simulink model "nav_flocking33"  (R2022b)
settings: Solver=FixedStepAuto  StartTime=0.0  StopTime=10.0  FixedStep=0.01  RelTol=1e-3
values from neighbouring files (symbols this model uses):
  a = 1    [main_flock3.m]    (also in main_flock4.m; params_flocking_ros.m)
  aR = diag([ar; ap; ay])    [main_flock3.m]    (also in main_flock4.m; main_sliding.m)
  Att1 = [2 -2 -15]    [main_flock3.m]    (also in main_flock4.m)
  Att2 = [2 -2 -15]    [main_flock3.m]    (also in main_flock4.m)
  Att3 = [2 -2 -15]    [main_flock3.m]    (also in main_flock4.m)
  b = 1    [main_flock3.m]    (also in main_flock4.m; params_flocking_ros.m)
  c = 1    [main_flock3.m]    (also in main_flock4.m; params_flocking_ros.m)
  c_gammap = 1.2    [main_flock3.m]    (also in main_flock4.m)
  c_gammav = 3.5    [main_flock3.m]    (also in main_flock4.m)
  d = 0.6    [main_flock3.m]    (also in main_flock4.m; params_flocking_ros.m)
  d_prime = 1    [main_flock3.m]    (also in main_flock4.m; params_flocking_ros.m)
  epsilon = 0.1    [main_flock3.m]    (also in main_flock4.m; params_flocking_ros.m)
  h = 0.2    [main_flock3.m]    (also in main_flock4.m; params_flocking_ros.m)
  K1 = diag([k111; k122; k133])    [main_flock3.m]    (also in main_flock4.m; main_sliding.m)
  K2 = diag([k211; k222; k233])    [main_flock3.m]    (also in main_flock4.m; main_sliding.m)
  Ki = diag([Ki1; Ki2; Ki3])    [main_flock3.m]    (also in main_flock4.m; main_sliding.m)
  lam = diag([lam1; lam2; lam3])    [main_flock3.m]    (also in main_flock4.m; main_sliding.m)
  R = 0.15    [main_flock3.m]    (also in main_flock4.m; params_flocking_ros.m)
  vxobs = 0    [main_flock3.m]    (also in main_flock4.m)
  vyobs = 0    [main_flock3.m]    (also in main_flock4.m)
  vzobs = 0    [main_flock3.m]    (also in main_flock4.m)
  X0_1 = [P01 dP01 om01]    [main_flock3.m]    (also in main_flock4.m; main_sliding.m = [P0 dP0 om0])
  X0_2 = [P02 dP02 om02]    [main_flock3.m]    (also in main_flock4.m)
  X0_3 = [P03 dP03 om03]    [main_flock3.m]    (also in main_flock4.m)
  xmax = 2    [main_flock3.m]    (also in main_flock4.m)
  xmin = -2    [main_flock3.m]    (also in main_flock4.m)
  xobs = 0.75    [main_flock3.m]    (also in main_flock4.m)
  yobs = -0.25    [main_flock3.m]    (also in main_flock4.m)
  zobs = 1.7    [main_flock3.m]    (also in main_flock4.m)
undefined symbols (not defined in the file or in its folder): A_Euler
libraries: aerosimlib x3
(part 2 of 2)

== matlab function nav_flocking33/Dron_dynamics2/Mixer (Parrot ARDRONE) ==
  data: T input; w1 output size=1; tau input; w2 output size=1; w3 output size=1; w4 output size=1
function [w1,w2,w3,w4]   = fcn(T, tau)
%#codegen
tau_phi = tau(1); 
tau_the = tau(2); 
tau_psi = tau(3);

% This values vary in fonction of the geometry of the drone 
b= 4.06e-6;
d= 7.5e-7;
l= (0.2)*(sin(pi/4));

%Parrot AR-DRONE 
uT = T/b; 
uphi = (sqrt(2)*tau_phi)/(b*l);  
uthe = (sqrt(2)*tau_the)/(b*l);
upsi = tau_psi/(d*l);

%Mix by Motors
mixM1 = uT+uphi-uthe+upsi;  %uT + for all mixM
mixM2 = uT-uphi-uthe-upsi; 
mixM3 = uT-uphi+uthe+upsi; 
mixM4 = uT+uphi+uthe-upsi;

%rotors speeds [rads/s]
w1= sign(mixM1)*sqrt(abs((1/4)*mixM1));
w2= sign(mixM2)*sqrt(abs((1/4)*mixM2));
w3= sign(mixM3)*sqrt(abs((1/4)*mixM3));
w4= sign(mixM4)*sqrt(abs((1/4)*mixM4));

== matlab function nav_flocking33/Subsystem2/Sliding mode (quaternions) ==
  data: qwe input; Gamma output; lam parameter; Ki parameter; K1 parameter; K2 parameter; aR parameter; s output
function [Gamma, s]  = fcn(qwe, lam, Ki, K1, K2, aR)

%Rotorcraft dimensions and parameters
Ix = 7.5e-3;
Iy = 7.5e-3;
Iz = 1.3e-2;

%Inertia
Ii=[Ix 0 0; 0 Iy 0; 0 0 Iz];

%Separation of rotational velocity and quaternion error in its components
qe = qwe(5:8);
qe1 = qe(1);
qe2 = qe(2);
qe3 = qe(3);
qe4 = qe(4);
qev = [qe2; qe3; qe4];

w = qwe(9:11);

iqe = qwe(12:15);
i_qe = [iqe(2); iqe(3); iqe(4)];

%Desired rotational velocity
wd = [0;0;0];

dwd = [0;0;0];

%Rotational velocity error in Euler
we = w - wd;
we1 = we(1);
we2 = we(2);
we3 = we(3);

%Quaternion error (derivative)
dqe0 = 0.5*(-we1*qe2 - we2*qe3 - we3*qe4);
dqe1 = 0.5*(we1*qe1 + we3*qe3 - we2*qe4);
dqe2 = 0.5*(we2*qe1 - we3*qe2 + we1*qe4);
dqe3 = 0.5*(we3*qe1 + we2*qe2 - we1*qe3);
dqe = [dqe1; dqe2; dqe3];

%Identity matrix
I3 = [1 0 0;
      0 1 0;
      0 0 1];
%Skew symmetrix matrix of vector part of the quaternion
sqev = [0 -qe4 qe3;
       qe4 0 -qe2;
       -qe3 qe2 0];
%ROTAION MATRIX: Given in Euler-Rodrigues formula
Re = (qe1^2 - qev'*qev)*I3 + 2*(qev*qev') - 2*qe1*sqev;

s = Ii*we + lam*qev + Ki*i_qe;

prod = cross(we,Re'*wd);

u = -lam*dqe - Ki*qev -Ii*(prod - Re'*dwd) + cross(w,Ii*w);       %Ks*qev

%Integral SMC 
Gamma = u - K1*tanh(inv(aR)*s) - K2*s;

== matlab function nav_flocking33/Translational Control2/Flocking1/MATLAB Function ==
  data: xi input; yi input; zi input; vxi input; vyi input; vzi input; phiAlpha output; aie output; aive output; xj input; yj input; zj input; vxj input; vyj input; vzj input; xk input; yk input; zk input; vxk input; vyk input; vzk input; epsilon parameter; a parameter; b parameter; c parameter; d parameter; e parameter; h parameter

function [phiAlpha, aie, aive]  = phiAlphaFcn(xi, yi, zi, vxi, vyi, vzi, xj, yj, zj, vxj, vyj, vzj, xk, yk, zk, vxk, vyk, vzk, epsilon, a, b, c, d, e, h)
    
    % Flocking parameters
    cAlpha = sigmaNormFun(c, epsilon) ;
    dAlpha = sigmaNormFun(d, epsilon) ;

    %%
    Pi = [xi;yi;zi] ;
    Pj = [xj;yj;zj] ;
    Pk = [xk;yk;zk] ;

    Vi = [vxi;vyi;vzi] ;
    Vj = [vxj;vyj;vzj] ;
    Vk = [vxk;vyk;vzk] ;
            
    %%
    sigmaNormj = sigmaNormFun(Pj - Pi, epsilon) ;
    nij = gradSigmaFun(Pj - Pi, epsilon) ;
    
    sigmaNormk = sigmaNormFun(Pk - Pi, epsilon) ;
    nik = gradSigmaFun(Pk - Pi, epsilon) ;

    %%
    sigma1j = sigma1Fun(sigmaNormj - dAlpha + e) ;
    sigma1k = sigma1Fun(sigmaNormk - dAlpha + e) ;
            
    %% Position
    phiAlphaj = 0.5 * bumpFcn(sigmaNormj/cAlpha,h) * ((a+b)*sigma1j + (a-b)) ;
    phiAlphanij = phiAlphaj.* nij ;
    
    phiAlphak = 0.5 * bumpFcn(sigmaNormk/cAlpha,h) * ((a+b)*sigma1k + (a-b)) ;
    phiAlphanik = phiAlphak.* nik ;

    phiAlpha = phiAlphanij + phiAlphanik;

    %
    aije = bumpFcn(sigmaNormj/cAlpha,h).*(Pj - Pi);

    aike = bumpFcn(sigmaNormj/cAlpha,h).*(Pk - Pi);

    aie = aije + aike;

    %% Velocity
    aijve = bumpFcn(sigmaNormj/cAlpha,h).*(Vj - Vi);

    aikve = bumpFcn(sigmaNormk/cAlpha,h).*(Vk - Vi);

    aive = aijve + aikve;
    
end

== matlab function nav_flocking33/Translational Control3/to_desired_angles ==
  data: Gamma input; cq_d output; Uz output
function [cq_d,Uz] = fcn(Gamma)

%Physical parameters
m = 0.65;
g = 9.81;

%Control signals separation
gamma = Gamma(1:3);
gamma1 = gamma(1);
gamma2 = gamma(2);
gamma3 = gamma(3);

%Desired Phi, theta, trust
psi = 0*pi/180;

phi = atan(gamma2/(gamma3+g));

theta = asin(-gamma1/(sqrt(gamma1^2+gamma2^2+(gamma3+g)^2)));

Uz = m*sqrt((gamma1)^2+(gamma2)^2+(gamma3+g)^2);

%Conversion to quaternions
q0 = cos(psi/2)*cos(theta/2)*cos(phi/2) + sin(psi/2)*sin(theta/2)*sin(phi/2);
q1 = cos(psi/2)*cos(theta/2)*sin(phi/2) - sin(psi/2)*sin(theta/2)*cos(phi/2);
q2 = cos(psi/2)*sin(theta/2)*cos(phi/2) + sin(psi/2)*cos(theta/2)*sin(phi/2);
q3 = sin(psi/2)*cos(theta/2)*cos(phi/2) - cos(psi/2)*sin(theta/2)*sin(phi/2);

cq_d = [q0;
        -q1;
        -q2;
        -q3];

== matlab function nav_flocking33/Translational Control1/Flocking1/MATLAB Function ==
  data: xi input; yi input; zi input; vxi input; vyi input; vzi input; phiAlpha output; aie output; aive output; xj input; yj input; zj input; vxj input; vyj input; vzj input; xk input; yk input; zk input; vxk input; vyk input; vzk input; epsilon parameter; a parameter; b parameter; c parameter; d parameter; e parameter; h parameter

function [phiAlpha, aie, aive]  = phiAlphaFcn(xi, yi, zi, vxi, vyi, vzi, xj, yj, zj, vxj, vyj, vzj, xk, yk, zk, vxk, vyk, vzk, epsilon, a, b, c, d, e, h)
    
    % Flocking parameters
    cAlpha = sigmaNormFun(c, epsilon) ;
    dAlpha = sigmaNormFun(d, epsilon) ;

    %%
    Pi = [xi;yi;zi] ;
    Pj = [xj;yj;zj] ;
    Pk = [xk;yk;zk] ;

    Vi = [vxi;vyi;vzi] ;
    Vj = [vxj;vyj;vzj] ;
    Vk = [vxk;vyk;vzk] ;
            
    %%
    sigmaNormj = sigmaNormFun(Pj - Pi, epsilon) ;
    nij = gradSigmaFun(Pj - Pi, epsilon) ;
    
    sigmaNormk = sigmaNormFun(Pk - Pi, epsilon) ;
    nik = gradSigmaFun(Pk - Pi, epsilon) ;

    %%
    sigma1j = sigma1Fun(sigmaNormj - dAlpha + e) ;
    sigma1k = sigma1Fun(sigmaNormk - dAlpha + e) ;
            
    %% Position
    phiAlphaj = 0.5 * bumpFcn(sigmaNormj/cAlpha,h) * ((a+b)*sigma1j + (a-b)) ;
    phiAlphanij = phiAlphaj.* nij ;
    
    phiAlphak = 0.5 * bumpFcn(sigmaNormk/cAlpha,h) * ((a+b)*sigma1k + (a-b)) ;
    phiAlphanik = phiAlphak.* nik ;

    phiAlpha = phiAlphanij + phiAlphanik;

    %
    aije = bumpFcn(sigmaNormj/cAlpha,h).*(Pj - Pi);

    aike = bumpFcn(sigmaNormj/cAlpha,h).*(Pk - Pi);

    aie = aije + aike;

    %% Velocity
    aijve = bumpFcn(sigmaNormj/cAlpha,h).*(Vj - Vi);

    aikve = bumpFcn(sigmaNormk/cAlpha,h).*(Vk - Vi);

    aive = aijve + aikve;
    
end

== matlab function nav_flocking33/Translational Control1/Flocking1/MATLAB Function1 ==
  data: phiAlpha input; phiAlpha_int input; aie input; aive input; ui_gamma input; phiBetak input; bikobs input; phiBetanei input; bikve input; Ui output size=3; KP parameter

function Ui  = ctrlLaw(phiAlpha, phiAlpha_int, aie, aive, ui_gamma, phiBetak, bikobs, phiBetanei, bikve, KP)  %, phiBetak, phiBetanei
    
    % Control gains and parameters
    Kx = KP(1); Ky = KP(2); Kz = KP(3);
    Kpx = KP(4); Kpy = KP(5); Kpz = KP(6);
    Kdx = KP(7); Kdy = KP(8); Kdz = KP(9);
    Kix = KP(10); Kiy = KP(11); Kiz = KP(12);
    cBetax = KP(13); cBetay = KP(14); cBetaz = KP(15);
    cdBetax = KP(16); cdBetay = KP(17); cdBetaz = KP(18);
    
        
    hx_dot = Kx * phiAlpha(1,1) + Kpx * aie(1,1) + Kdx * aive(1,1) + Kix * phiAlpha_int(1,1) + ui_gamma(1,1) + cBetax * (phiBetak(1,1) + phiBetanei(1,1)) + cdBetax * (bikobs(1,1) + bikve(1,1));
    hy_dot = Ky * phiAlpha(2,1) + Kpy * aie(2,1) + Kdy * aive(2,1) + Kiy * phiAlpha_int(2,1) + ui_gamma(2,1) + cBetay * (phiBetak(2,1) + phiBetanei(2,1)) + cdBetay * (bikobs(2,1) + bikve(2,1));
    hz_dot = Kz * phiAlpha(3,1) + Kpz * aie(3,1) + Kdz * aive(3,1) + Kiz * phiAlpha_int(3,1) + ui_gamma(3,1) + cBetaz * (phiBetak(3,1) + phiBetanei(3,1)) + cdBetaz * (bikobs(3,1) + bikve(3,1));
    

    Ui = [hx_dot; hy_dot; hz_dot] ;
        
end

== matlab function nav_flocking33/Translational Control1/Flocking1/MATLAB Function2 ==
  data: xi input; yi input; zi input; vxi input; vyi input; vzi input; ui_gamma output; xr input; yr input; zr input; vxr input; vyr input; vzr input; c_gammap parameter; xmin parameter; xmax parameter; c_gammav parameter

function ui_gamma   = naviFeedback(xi, yi, zi, vxi, vyi, vzi, xr, yr, zr, vxr, vyr, vzr, c_gammap, xmin, xmax, c_gammav)
    
       
    Pi = [xi ; yi ; zi] ;
    Vi = [vxi ; vyi ; vzi] ;


    Pr = [xr ; yr ; zr] ;
    Vr = [vxr ; vyr ; vzr] ;
    
    ui_gamma = (-1).* satFcn(c_gammap.*(Pi - Pr), xmin, xmax) + (-1).* satFcn(c_gammav.*(Vi - Vr), xmin, xmax) ;
    
end

== matlab function nav_flocking33/Translational Control1/Flocking1/MATLAB Function3 ==
  data: xi input; yi input; zi input; vxi input; vyi input; vzi input; xobs parameter; yobs parameter; zobs parameter; vxobs parameter; vyobs parameter; vzobs parameter; phiBetanik output; R parameter; epsilon parameter; d_prime parameter; h parameter; bikobs output
function [phiBetanik, bikobs] = phiBetaFcn(xi, yi, zi, vxi, vyi, vzi, xobs, yobs, zobs, vxobs, vyobs, vzobs, R, epsilon, d_prime, h)
    
    dBeta = sigmaNormFun(d_prime, epsilon) ;
    
    Pi = [xi ; yi ; zi] ;
    Pc = [xobs ; yobs ; zobs] ;
    
    Vi = [vxi ; vyi ; vzi] ;
    Vc = [vxobs ; vyobs ; vzobs] ;

    % Compute closest point between the robot center and the obstacle
    % circumference (ossumming obstacles are circles)
    Pk = Pc + (Pi - Pc) * (R /norm(Pi - Pc)) ;
    %Pk = [xobs ; yobs] ;
    
    sigmaNormk = sigmaNormFun(Pk - Pi, epsilon) ;
    nik = gradSigmaFun(Pk - Pi, epsilon) ;
    
    sigma1k = sigma1Fun(sigmaNormk - dBeta) ;
    
    %% Position
    phiBetak = bumpFcn(sigmaNormk/dBeta,h) * (sigma1k - 1) ;
    phiBetanik = phiBetak.* nik ;
    
    %% Velocity
    bikobs = bumpFcn(sigmaNormk/dBeta,h).*(Vc + (Vi - Vc));
end

== matlab function nav_flocking33/Translational Control1/Flocking1/MATLAB Function4 ==
  data: xj input; yj input; zj input; vxj input; vyj input; vzj input; xk input; yk input; zk input; vxk input; vyk input; vzk input; xobs parameter; yobs parameter; zobs parameter; phiBetaniknei output; R parameter; epsilon parameter; d_prime parameter; h parameter; vxobs parameter; vyobs parameter; vzobs parameter; bikve output
function [phiBetaniknei, bikve] = phiBetaFcn(xj, yj, zj, vxj, vyj, vzj, xk, yk, zk, vxk, vyk, vzk, xobs, yobs, zobs, R, epsilon, d_prime, h, vxobs, vyobs, vzobs)
    
    dBeta = sigmaNormFun(d_prime, epsilon) ;
    
    Pj = [xj ; yj ; zj] ;
    Pk = [xk ; yk ; zk] ;
    Pc = [xobs ; yobs ; zobs] ;

    Vj = [vxj ; vyj ; vzj] ;
    Vk = [vxk ; vyk ; vzk] ;
    Vc = [vxobs ; vyobs ; vzobs] ;

    % Compute closest point between the robot center and the obstacle
    % circumference (ossumming obstacles are circles)
    Pobsj = Pc + (Pj - Pc) * (R /norm(Pj - Pc)) ;
    Pobsk = Pc + (Pk - Pc) * (R /norm(Pk - Pc)) ;
    %Pk = [xobs ; yobs] ;
    
    %%
    sigmaNormj = sigmaNormFun(Pobsj - Pj, epsilon) ;
    nij = gradSigmaFun(Pobsj - Pj, epsilon) ;
    
    sigmaNormk = sigmaNormFun(Pobsk - Pk, epsilon) ;
    nik = gradSigmaFun(Pobsk - Pk, epsilon) ;

    %%
    sigma1j = sigma1Fun(sigmaNormj - dBeta) ;
    sigma1k = sigma1Fun(sigmaNormk - dBeta) ;
            
    %%
    phiBetaj = bumpFcn(sigmaNormj/dBeta,h) * (sigma1j - 1) ;
    phiBetak = bumpFcn(sigmaNormk/dBeta,h) * (sigma1k - 1) ;
            
    %% Position
    phiBetaniknei = phiBetaj.* nij + phiBetak.* nik;
    
    %% Velocity
    bikve = bumpFcn(sigmaNormj/dBeta,h).*(Vc + (Vj - Vc)) + bumpFcn(sigmaNormk/dBeta,h).*(Vc + (Vk - Vc));
end

== matlab function nav_flocking33/Translational Control3/Flocking1/MATLAB Function2 ==
  data: xi input; yi input; zi input; vxi input; vyi input; vzi input; ui_gamma output; xr input; yr input; zr input; vxr input; vyr input; vzr input; c_gammap parameter; xmin parameter; xmax parameter; c_gammav parameter

function ui_gamma   = naviFeedback(xi, yi, zi, vxi, vyi, vzi, xr, yr, zr, vxr, vyr, vzr, c_gammap, xmin, xmax, c_gammav)
    
       
    Pi = [xi ; yi ; zi] ;
    Vi = [vxi ; vyi ; vzi] ;


    Pr = [xr ; yr ; zr] ;
    Vr = [vxr ; vyr ; vzr] ;
    
    ui_gamma = (-1).* satFcn(c_gammap.*(Pi - Pr), xmin, xmax) + (-1).* satFcn(c_gammav.*(Vi - Vr), xmin, xmax) ;
    
end

== matlab function nav_flocking33/Translational Control2/Flocking1/MATLAB Function1 ==
  data: phiAlpha input; phiAlpha_int input; aie input; aive input; ui_gamma input; phiBetak input; bikobs input; phiBetanei input; bikve input; Ui output size=3; KP parameter

function Ui  = ctrlLaw(phiAlpha, phiAlpha_int, aie, aive, ui_gamma, phiBetak, bikobs, phiBetanei, bikve, KP)  %, phiBetak, phiBetanei
    
    % Control gains and parameters
    Kx = KP(1); Ky = KP(2); Kz = KP(3);
    Kpx = KP(4); Kpy = KP(5); Kpz = KP(6);
    Kdx = KP(7); Kdy = KP(8); Kdz = KP(9);
    Kix = KP(10); Kiy = KP(11); Kiz = KP(12);
    cBetax = KP(13); cBetay = KP(14); cBetaz = KP(15);
    cdBetax = KP(16); cdBetay = KP(17); cdBetaz = KP(18);
    
        
    hx_dot = Kx * phiAlpha(1,1) + Kpx * aie(1,1) + Kdx * aive(1,1) + Kix * phiAlpha_int(1,1) + ui_gamma(1,1) + cBetax * (phiBetak(1,1) + phiBetanei(1,1)) + cdBetax * (bikobs(1,1) + bikve(1,1));
    hy_dot = Ky * phiAlpha(2,1) + Kpy * aie(2,1) + Kdy * aive(2,1) + Kiy * phiAlpha_int(2,1) + ui_gamma(2,1) + cBetay * (phiBetak(2,1) + phiBetanei(2,1)) + cdBetay * (bikobs(2,1) + bikve(2,1));
    hz_dot = Kz * phiAlpha(3,1) + Kpz * aie(3,1) + Kdz * aive(3,1) + Kiz * phiAlpha_int(3,1) + ui_gamma(3,1) + cBetaz * (phiBetak(3,1) + phiBetanei(3,1)) + cdBetaz * (bikobs(3,1) + bikve(3,1));
    

    Ui = [hx_dot; hy_dot; hz_dot] ;
        
end

== matlab function nav_flocking33/Translational Control2/Flocking1/MATLAB Function2 ==
  data: xi input; yi input; zi input; vxi input; vyi input; vzi input; ui_gamma output; xr input; yr input; zr input; vxr input; vyr input; vzr input; c_gammap parameter; xmin parameter; xmax parameter; c_gammav parameter

function ui_gamma   = naviFeedback(xi, yi, zi, vxi, vyi, vzi, xr, yr, zr, vxr, vyr, vzr, c_gammap, xmin, xmax, c_gammav)
    
       
    Pi = [xi ; yi ; zi] ;
    Vi = [vxi ; vyi ; vzi] ;


    Pr = [xr ; yr ; zr] ;
    Vr = [vxr ; vyr ; vzr] ;
    
    ui_gamma = (-1).* satFcn(c_gammap.*(Pi - Pr), xmin, xmax) + (-1).* satFcn(c_gammav.*(Vi - Vr), xmin, xmax) ;
    
end

== matlab function nav_flocking33/Translational Control2/Flocking1/MATLAB Function3 ==
  data: xi input; yi input; zi input; vxi input; vyi input; vzi input; xobs parameter; yobs parameter; zobs parameter; vxobs parameter; vyobs parameter; vzobs parameter; phiBetanik output; R parameter; epsilon parameter; d_prime parameter; h parameter; bikobs output
function [phiBetanik, bikobs] = phiBetaFcn(xi, yi, zi, vxi, vyi, vzi, xobs, yobs, zobs, vxobs, vyobs, vzobs, R, epsilon, d_prime, h)
    
    dBeta = sigmaNormFun(d_prime, epsilon) ;
    
    Pi = [xi ; yi ; zi] ;
    Pc = [xobs ; yobs ; zobs] ;
    
    Vi = [vxi ; vyi ; vzi] ;
    Vc = [vxobs ; vyobs ; vzobs] ;

    % Compute closest point between the robot center and the obstacle
    % circumference (ossumming obstacles are circles)
    Pk = Pc + (Pi - Pc) * (R /norm(Pi - Pc)) ;
    %Pk = [xobs ; yobs] ;
    
    sigmaNormk = sigmaNormFun(Pk - Pi, epsilon) ;
    nik = gradSigmaFun(Pk - Pi, epsilon) ;
    
    sigma1k = sigma1Fun(sigmaNormk - dBeta) ;
    
    %% Position
    phiBetak = bumpFcn(sigmaNormk/dBeta,h) * (sigma1k - 1) ;
    phiBetanik = phiBetak.* nik ;
    
    %% Velocity
    bikobs = bumpFcn(sigmaNormk/dBeta,h).*(Vc + (Vi - Vc));
end

== matlab function nav_flocking33/Translational Control2/Flocking1/MATLAB Function4 ==
  data: xj input; yj input; zj input; vxj input; vyj input; vzj input; xk input; yk input; zk input; vxk input; vyk input; vzk input; xobs parameter; yobs parameter; zobs parameter; phiBetaniknei output; R parameter; epsilon parameter; d_prime parameter; h parameter; vxobs parameter; vyobs parameter; vzobs parameter; bikve output
function [phiBetaniknei, bikve] = phiBetaFcn(xj, yj, zj, vxj, vyj, vzj, xk, yk, zk, vxk, vyk, vzk, xobs, yobs, zobs, R, epsilon, d_prime, h, vxobs, vyobs, vzobs)
    
    dBeta = sigmaNormFun(d_prime, epsilon) ;
    
    Pj = [xj ; yj ; zj] ;
    Pk = [xk ; yk ; zk] ;
    Pc = [xobs ; yobs ; zobs] ;

    Vj = [vxj ; vyj ; vzj] ;
    Vk = [vxk ; vyk ; vzk] ;
    Vc = [vxobs ; vyobs ; vzobs] ;

    % Compute closest point between the robot center and the obstacle
    % circumference (ossumming obstacles are circles)
    Pobsj = Pc + (Pj - Pc) * (R /norm(Pj - Pc)) ;
    Pobsk = Pc + (Pk - Pc) * (R /norm(Pk - Pc)) ;
    %Pk = [xobs ; yobs] ;
    
    %%
    sigmaNormj = sigmaNormFun(Pobsj - Pj, epsilon) ;
    nij = gradSigmaFun(Pobsj - Pj, epsilon) ;
    
    sigmaNormk = sigmaNormFun(Pobsk - Pk, epsilon) ;
    nik = gradSigmaFun(Pobsk - Pk, epsilon) ;

    %%
    sigma1j = sigma1Fun(sigmaNormj - dBeta) ;
    sigma1k = sigma1Fun(sigmaNormk - dBeta) ;
            
    %%
    phiBetaj = bumpFcn(sigmaNormj/dBeta,h) * (sigma1j - 1) ;
    phiBetak = bumpFcn(sigmaNormk/dBeta,h) * (sigma1k - 1) ;
            
    %% Position
    phiBetaniknei = phiBetaj.* nij + phiBetak.* nik;
    
    %% Velocity
    bikve = bumpFcn(sigmaNormj/dBeta,h).*(Vc + (Vj - Vc)) + bumpFcn(sigmaNormk/dBeta,h).*(Vc + (Vk - Vc));
end

== matlab function nav_flocking33/Translational Control3/Flocking1/MATLAB Function3 ==
  data: xi input; yi input; zi input; vxi input; vyi input; vzi input; xobs parameter; yobs parameter; zobs parameter; vxobs parameter; vyobs parameter; vzobs parameter; phiBetanik output; R parameter; epsilon parameter; d_prime parameter; h parameter; bikobs output
function [phiBetanik, bikobs] = phiBetaFcn(xi, yi, zi, vxi, vyi, vzi, xobs, yobs, zobs, vxobs, vyobs, vzobs, R, epsilon, d_prime, h)
    
    dBeta = sigmaNormFun(d_prime, epsilon) ;
    
    Pi = [xi ; yi ; zi] ;
    Pc = [xobs ; yobs ; zobs] ;
    
    Vi = [vxi ; vyi ; vzi] ;
    Vc = [vxobs ; vyobs ; vzobs] ;

    % Compute closest point between the robot center and the obstacle
    % circumference (ossumming obstacles are circles)
    Pk = Pc + (Pi - Pc) * (R /norm(Pi - Pc)) ;
    %Pk = [xobs ; yobs] ;
    
    sigmaNormk = sigmaNormFun(Pk - Pi, epsilon) ;
    nik = gradSigmaFun(Pk - Pi, epsilon) ;
    
    sigma1k = sigma1Fun(sigmaNormk - dBeta) ;
    
    %% Position
    phiBetak = bumpFcn(sigmaNormk/dBeta,h) * (sigma1k - 1) ;
    phiBetanik = phiBetak.* nik ;
    
    %% Velocity
    bikobs = bumpFcn(sigmaNormk/dBeta,h).*(Vc + (Vi - Vc));
end

== matlab function nav_flocking33/Translational Control3/Flocking1/MATLAB Function4 ==
  data: xj input; yj input; zj input; vxj input; vyj input; vzj input; xk input; yk input; zk input; vxk input; vyk input; vzk input; xobs parameter; yobs parameter; zobs parameter; phiBetaniknei output; R parameter; epsilon parameter; d_prime parameter; h parameter; vxobs parameter; vyobs parameter; vzobs parameter; bikve output
function [phiBetaniknei, bikve] = phiBetaFcn(xj, yj, zj, vxj, vyj, vzj, xk, yk, zk, vxk, vyk, vzk, xobs, yobs, zobs, R, epsilon, d_prime, h, vxobs, vyobs, vzobs)
    
    dBeta = sigmaNormFun(d_prime, epsilon) ;
    
    Pj = [xj ; yj ; zj] ;
    Pk = [xk ; yk ; zk] ;
    Pc = [xobs ; yobs ; zobs] ;

    Vj = [vxj ; vyj ; vzj] ;
    Vk = [vxk ; vyk ; vzk] ;
    Vc = [vxobs ; vyobs ; vzobs] ;

    % Compute closest point between the robot center and the obstacle
    % circumference (ossumming obstacles are circles)
    Pobsj = Pc + (Pj - Pc) * (R /norm(Pj - Pc)) ;
    Pobsk = Pc + (Pk - Pc) * (R /norm(Pk - Pc)) ;
    %Pk = [xobs ; yobs] ;
    
    %%
    sigmaNormj = sigmaNormFun(Pobsj - Pj, epsilon) ;
    nij = gradSigmaFun(Pobsj - Pj, epsilon) ;
    
    sigmaNormk = sigmaNormFun(Pobsk - Pk, epsilon) ;
    nik = gradSigmaFun(Pobsk - Pk, epsilon) ;

    %%
    sigma1j = sigma1Fun(sigmaNormj - dBeta) ;
    sigma1k = sigma1Fun(sigmaNormk - dBeta) ;
            
    %%
    phiBetaj = bumpFcn(sigmaNormj/dBeta,h) * (sigma1j - 1) ;
    phiBetak = bumpFcn(sigmaNormk/dBeta,h) * (sigma1k - 1) ;
            
    %% Position
    phiBetaniknei = phiBetaj.* nij + phiBetak.* nik;
    
    %% Velocity
    bikve = bumpFcn(sigmaNormj/dBeta,h).*(Vc + (Vj - Vc)) + bumpFcn(sigmaNormk/dBeta,h).*(Vc + (Vk - Vc));
end

== matlab function nav_flocking33/Dron_dynamics/MATLAB Function1 ==
  data: X input; dX output; X2 input; dotq output; as input
function [dX,dotq] = fcn(X, X2, as)
% Jonatan Alvarez / October 2021
% Rotorcraft 3D Model (based on the quaternion parametrization) 

%Rotorcraft dimensions and parameters
m=0.65;   
g = 9.81;
Ix = 7.5e-3;
Iy = 7.5e-3;
Iz = 1.3e-2;
e  = 4.06e-6;
d  = 7.5e-7;
l  = (0.2)*(sin(pi/4));

%Inertia
Ii=[Ix 0 0; 0 Iy 0; 0 0 Iz];

%Extraction of data
x = X(1:3);
dx = X(4:6);
om = X(7:9); %Angular velocity

%Wind


%Separation of the angular velocity and quaternions in its components
om1 = om(1);
om2 = om(2);
om3 = om(3);

q = X2(1:4);
q1 = q(1);
q2 = q(2);
q3 = q(3);
q4 = q(4);
qv = [q2;q3;q4];

%EXTRACTION OF ROTOR SPEEDS AND FORCES COMPUTATION
u = as(1:4);
%Motor forces (e3)
f1= e*u(1)^2; f2=e*u(2)^2;  f3=e*u(3)^2; f4=e*u(4)^2; % rotors' blades lift forces
f1d = d*u(1)^2; f2d=d*u(2)^2;  f3d=d*u(3)^2; f4d=d*u(4)^2; %rotors' blades drag forces
%Torques
tau_phi = (1/sqrt(2))*l*(f1-f2-f3+f4) ;
tau_the = (1/sqrt(2))*l*(-f1-f2+f3+f4);
tau_psi = l*(f1d-f2d+f3d-f4d);
%MAIN Thrust and Torque vectors
Th =[0;0;f1+f2+f3+f4];
F = [tau_phi;tau_the;tau_psi];

%ROTATIONAL MOTION
%Quaternions
dq0 = 0.5*(-om1*q2 - om2*q3 - om3*q4);
dq1 = 0.5*(om1*q1 + om3*q3 - om2*q4);
dq2 = 0.5*(om2*q1 - om3*q2 + om1*q4);
dq3 = 0.5*(om3*q1 + om2*q2 - om1*q3);
%Attitude kinematics in quaternions
dotq = [dq0;dq1;dq2;dq3];  
%Attitude dynamics
dW =  inv(Ii)*( - cross(om,Ii*om) + F);

%TRANSLATIONAL MOTION
%Identity matrix
I3 = [1 0 0;
      0 1 0;
      0 0 1];
%Skew symmetrix matrix of vector part of the quaternion
sqv = [0 -q4 q3;
       q4 0 -q2;
       -q3 q2 0];
%Rotation matrix: given in Euler-Rodrigues formula
R = (q1^2 - qv'*qv)*I3 + 2*(qv*qv') - 2*q1*sqv;
%R = I3 - 2*q1*(sqv) + 2*(sqv)^2;
%Mass matrix
M_xi=[m  0  0;
      0  m  0;
      0  0  m];
%Vector fo Gravitational terms and thrust
G_xi=[0;0;m*g];
%Th = [0;0;T];
%Linear dynamics
Ddx =  inv(M_xi)*( -G_xi + R*Th);  % +fa

%Final vector
dX = [dx;Ddx;dW];

== matlab function nav_flocking33/Dron_dynamics/Mixer (Parrot ARDRONE) ==
  data: T input; w1 output size=1; tau input; w2 output size=1; w3 output size=1; w4 output size=1
function [w1,w2,w3,w4]   = fcn(T, tau)
%#codegen
tau_phi = tau(1); 
tau_the = tau(2); 
tau_psi = tau(3);

% This values vary in fonction of the geometry of the drone 
b= 4.06e-6;
d= 7.5e-7;
l= (0.2)*(sin(pi/4));

%Parrot AR-DRONE 
uT = T/b; 
uphi = (sqrt(2)*tau_phi)/(b*l);  
uthe = (sqrt(2)*tau_the)/(b*l);
upsi = tau_psi/(d*l);

%Mix by Motors
mixM1 = uT+uphi-uthe+upsi;  %uT + for all mixM
mixM2 = uT-uphi-uthe-upsi; 
mixM3 = uT-uphi+uthe+upsi; 
mixM4 = uT+uphi+uthe-upsi;

%rotors speeds [rads/s]
w1= sign(mixM1)*sqrt(abs((1/4)*mixM1));
w2= sign(mixM2)*sqrt(abs((1/4)*mixM2));
w3= sign(mixM3)*sqrt(abs((1/4)*mixM3));
w4= sign(mixM4)*sqrt(abs((1/4)*mixM4));

== matlab function nav_flocking33/Virtual_leader ==
  data: t input; xi_d output; dxi_d output; ddxi_d output
function [xi_d, dxi_d, ddxi_d]  = fcn(t)
%#codegen

f=1/14;    %freq in Hz
radius=2;   %radius in meters
f2 = 1/35;
radius2 = 1;
sel=1;      %inputs or parameters dont work! only local vars ...

if sel == 1
    if t < 20
       xd     =  0;
       xdotd  =  0;
       xddotd =  0;   
    
       yd     = 0;
       ydotd  = 0;
       yddotd = 0;
    
       zd     = 1.5;  
       zdotd  = 0; 
       zddotd = 0;
    
       xi_d =[xd; yd; zd];
       dxi_d=[xdotd; ydotd; zdotd]; 
       ddxi_d = [xddotd; yddotd; zddotd];
    elseif t < 40
        xd     =  1.5;
        xdotd  =  0;
        xddotd =  0;   
    
        yd     = -1.5;
        ydotd  = 0;
        yddotd = 0;
    
        zd     = 2;  
        zdotd  = 0; 
        zddotd = 0;
    
        xi_d =[xd; yd; zd];
        dxi_d=[xdotd; ydotd; zdotd]; 
        ddxi_d = [xddotd; yddotd; zddotd];
    else
       xd     = radius*sin(2*pi*f*t);
       xdotd  = radius*2*pi*f*cos(2*pi*f*t);
       xddotd = -radius*4*pi^2*f^2*sin(2*pi*f*t);
     
       yd     = radius*cos(2*pi*f*t);
       ydotd  = -radius*2*pi*f*sin(2*pi*f*t);
       yddotd =  -radius*4*pi^2*f^2*cos(2*pi*f*t);0;
     
       zd     = 3;  %radius*cos(2*pi*f*t) + 5;
       zdotd  = 0;  %-radius*2*pi*f*sin(2*pi*f*t);
       zddotd = 0;  %-radius*4*pi^2*f^2*cos(2*pi*f*t);
    
       xi_d =[xd; yd; zd];
       dxi_d=[xdotd; ydotd; zdotd];
       ddxi_d = [xddotd; yddotd; zddotd];
    end
end

 if(sel==2)
     xd     =  0;
     xdotd  =  0;
     xddotd =  0;   
     
     yd     = 0;
     ydotd  = 0;
     yddotd = 0;
     
     zd     = 1.5;  
     zdotd  = 0; 
     zddotd = 0;
     
     xi_d =[xd; yd; zd];
     dxi_d=[xdotd; ydotd; zdotd]; 
     ddxi_d = [xddotd; yddotd; zddotd];
 end
